simulink model "sm_control_feedback"  (R2016a)
settings: Solver=VariableStepAuto  StartTime=0.0  StopTime=10.0  RelTol=1e-3
libraries: powerlib x12, simulink x1
settings Model: Creator=jorda  LastModifiedBy=jorda

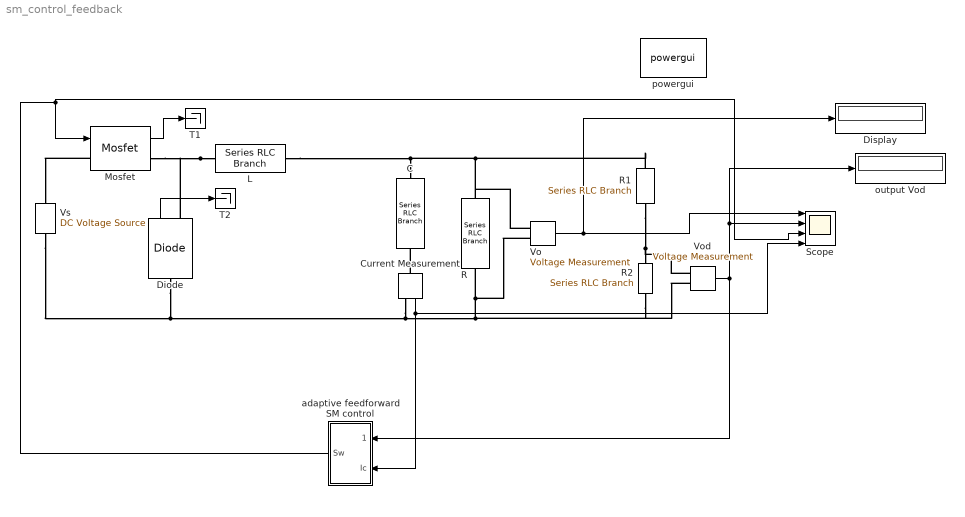
== system sm_control_feedback ==
  C : powerlib/Elements/Series RLC Branch  LConnTagsString=__new0  RConnTagsString=__new0  BranchType=C  Resistance=1  Inductance=1e-3  SetiL0=off  InitialCurrent=0  Capacitance=2000e-6  Setx0=off  InitialVoltage=0  Measurements=None
  Current Measurement : powerlib/Measurements/Current Measurement  PhasorSimulation=off  OutputType=Complex  PSBequivalent=0
  Diode : powerlib/Power Electronics/Diode  Ron=0.001  Lon=0  Vf=0.8  IC=0  UseSnubber=off  Rs=500  Cs=250e-9  Measurements=on
  Display : Display
  L : powerlib/Elements/Series RLC Branch  LConnTagsString=__new0  RConnTagsString=__new0  BranchType=L  Resistance=1  Inductance=2e-3  SetiL0=off  InitialCurrent=0  Capacitance=1e-6  Setx0=off  InitialVoltage=0  Measurements=None
  Mosfet : powerlib/Power Electronics/Mosfet  Ron=0.1  Lon=0  Rd=0.01  Vfd=0  IC=0  Rs=1e5  Cs=inf  Measurements=on
  R : powerlib/Elements/Series RLC Branch  LConnTagsString=__new0  RConnTagsString=__new0  BranchType=R  Resistance=4  Inductance=1e-3  SetiL0=off  InitialCurrent=0  Capacitance=1e-6  Setx0=off  InitialVoltage=0  Measurements=None
  R1 : powerlib/Elements/Series RLC Branch  LConnTagsString=__new0  RConnTagsString=__new0  BranchType=R  Resistance=317  Inductance=1e-3  SetiL0=off  InitialCurrent=0  Capacitance=1e-6  Setx0=off  InitialVoltage=0  Measurements=None
  R2 : powerlib/Elements/Series RLC Branch  LConnTagsString=__new0  RConnTagsString=__new0  BranchType=R  Resistance=870  Inductance=1e-3  SetiL0=off  InitialCurrent=0  Capacitance=1e-6  Setx0=off  InitialVoltage=0  Measurements=None
  Scope : Scope  NumInputPorts=4
  T1 : Terminator
  T2 : Terminator
  Vo : powerlib/Measurements/Voltage Measurement  PhasorSimulation=off  OutputType=Complex  PSBequivalent=0
  Vod : powerlib/Measurements/Voltage Measurement  PhasorSimulation=off  OutputType=Complex  PSBequivalent=0
  Vs : powerlib/Electrical Sources/DC Voltage Source  Amplitude=15  Measurements=None
  adaptive feedforward SM control : Subsystem
  output Vod : Display
  powergui : powerlib/powergui  Priority=1  SimulationMode=Continuous  SolverType=Tustin/Backward Euler (TBE)  SampleTime=50e-6  frequency=60  SPID=off  DisableSnubberDevices=off  DisableRonSwitches=off  DisableVfSwitches=off  SwTol=0  DisplayEquations=off  Interpol=off  ExternalGateDelay=off  methode=off  Ts=10  FunctionMessages=off  echomessages=off  HookPort=off  EnableUseOfTLC=off  x0status=blocks  frequencyindice=60  Pbase=100e6  ErrMax=1e-4  Iterations=50  UnitsV=kV  UnitsW=MW  buscounter=0  RestoreLinks=warning  ResistiveCurrentMeasurement=off  Frange=[0:2:500]  Ylog=off  Xlog=on  ShowGrid=off  save=off  variable=ZData  structure=0  ZoomFFT=off  StartTime=0.0  cycles=1  DisplayStyle=1  fundamental=60  FreqAxis=off  MaxFrequency=1000  frequencyindicesteady=1  RmsSteady=1  display=off
  wires:
  Diode/1 -> T2/1
  Mosfet/1 -> T1/1
  Current Measurement/1 -> Scope/4, adaptive feedforward SM control/2(Ic)
  adaptive feedforward SM control/1(Sw) -> Mosfet/1, Scope/3
  Vod/1 -> adaptive feedforward SM control/1(Vod), Scope/2, output Vod/1
  Vo/1 -> Display/1, Scope/1
  connections:
  R1/LConn1 -- L/RConn1 -- C/LConn1 -- R/LConn1 -- Vo/LConn1
  Diode/LConn1 -- Vs/LConn1 -- Current Measurement/RConn1 -- R2/RConn1 -- Vod/LConn2 -- R/RConn1 -- Vo/LConn2
  L/LConn1 -- Mosfet/RConn1 -- Diode/RConn1
  R2/LConn1 -- R1/RConn1 -- Vod/LConn1
  Current Measurement/LConn1 -- C/RConn1
  Mosfet/LConn1 -- Vs/RConn1

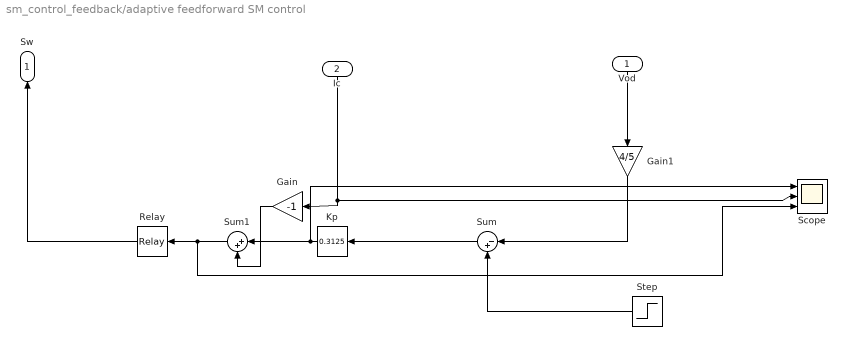
== system sm_control_feedback/adaptive feedforward SM control ==
  Vod : Inport
  Ic : Inport  Port=2
  Gain : Gain  Gain=-1  ParamDataTypeStr=double  OutDataTypeStr=double
  Gain1 : Gain  Gain=4/5  ParamDataTypeStr=double  OutDataTypeStr=double
  Kp : simulink/Math Operations/Slider Gain  low=0  gain=0.3125  high=8000
  Relay : Relay  OnSwitchValue=0.833  OffSwitchValue=-0.833  OutDataTypeStr=Inherit: Inherit via back propagation
  Scope : Scope  NumInputPorts=3
  Step : Step  Time=0  Before=4  After=4  SampleTime=0
  Sum : Sum  Inputs=|-+  AccumDataTypeStr=single  OutDataTypeStr=double  InputSameDT=on
  Sum1 : Sum  Inputs=|++  AccumDataTypeStr=double  OutDataTypeStr=double  InputSameDT=on
  Sw : Outport
  wires:
  Gain1/1 -> Sum/1
  Ic/1 -> Scope/2, Gain/1
  Vod/1 -> Gain1/1
  Step/1 -> Sum/2
  Sum1/1 -> Scope/3, Relay/1
  Kp/1 -> Sum1/1, Scope/1
  Sum/1 -> Kp/1
  Gain/1 -> Sum1/2
  Relay/1 -> Sw/1
